simulink model "filter_direct"  (R2020a)
settings: Solver=FixedStepAuto  StartTime=0.0  StopTime=10.0  FixedStep=0.2  RelTol=1e-3
settings Model: Creator=kiran  LastModifiedBy=kiran
settings DataIOCC: SaveOutput=off  SaveTime=off

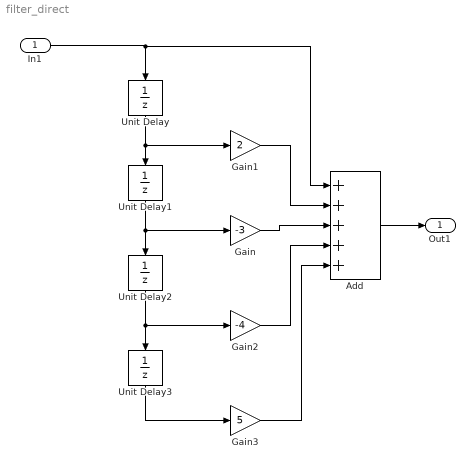
== system filter_direct ==
  In1 : Inport  OutDataTypeStr=double  PortDimensions=1  SampleTime=[0.20000000000000001,0]
  Add : Sum  Inputs=+++++
  Gain : Gain  Gain=-3
  Gain1 : Gain  Gain=2
  Gain2 : Gain  Gain=-4
  Gain3 : Gain  Gain=5
  Unit Delay{,1..3} (4 alike) : UnitDelay  SampleTime=-1  HasFrameUpgradeWarning=on
  Out1 : Outport  OutDataTypeStr=double  PortDimensions=1  SampleTime=[0.20000000000000001,0]
  wires:
  Gain1/1 -> Add/2
  Gain3/1 -> Add/5
  Gain2/1 -> Add/4
  Unit Delay1/1 -> Gain/1, Unit Delay2/1
  Gain/1 -> Add/3
  Unit Delay3/1 -> Gain3/1
  Unit Delay2/1 -> Unit Delay3/1, Gain2/1
  In1/1 -> Unit Delay/1, Add/1
  Unit Delay/1 -> Gain1/1, Unit Delay1/1
  Add/1 -> Out1/1
